simulink model "Example1"  (R2015a)
settings: Solver=ode45  StartTime=0.0  StopTime=10.0  RelTol=1e-3
settings Model: Creator=Suwandi Dwi S  LastModifiedBy=Suwandi Dwi S

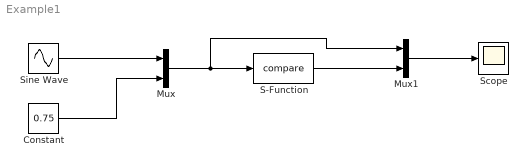
== system Example1 ==
  Constant : Constant  Value=0.75
  Mux : Mux  Inputs=2
  Mux1 : Mux  Inputs=2
  S-Function : S-Function  FunctionName=compare
  Scope : Scope
  Sine Wave : Sin  SampleTime=0
  wires:
  Mux/1 -> S-Function/1, Mux1/1
  S-Function/1 -> Mux1/2
  Mux1/1 -> Scope/1
  Sine Wave/1 -> Mux/1
  Constant/1 -> Mux/2
